simulink library "HeatSourceControl"  (R2025a)
settings: Solver=VariableStepAuto  StartTime=0.0  StopTime=10.0  RelTol=1e-3
libraries: fl_lib x11
settings Model: Creator=vikrants  LastModifiedBy=vikrants

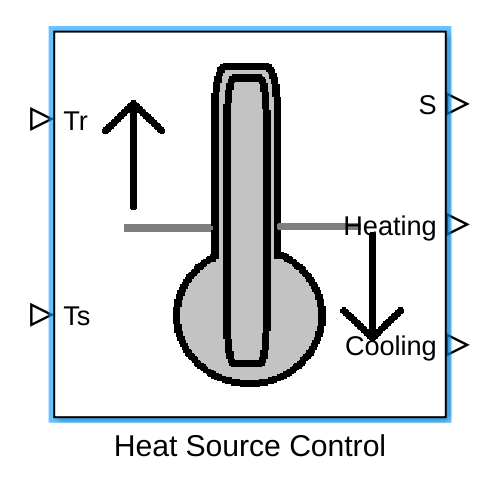
[thumbnail: Simulink's stored preview of the top-level diagram]
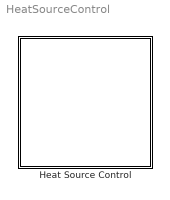
== system HeatSourceControl ==
  Heat Source Control : Subsystem  mask{capacity=12000, num=1, delT=10, tau=1, iniT=280}
      mask prompts: capacity "Heat pump capacity (W)"; num "Number of sources (-)"; delT "Change in water temperature (deg C)"; tau "Measurement time constant (s)"; iniT "Initial water temperature (K)"
      mask Help: web("DocumentationCompositeHeatSourceControl.html")
      mask DialogControl DescGroupVar Prompt: Description
      mask DialogControl DescTextVar Prompt: The block evaluates heating or cooling requirements for a building  based on the measured room temperatures and the specified set point temperature.
      mask DialogControl HeatPump Prompt: Heat Pump
      mask Display: image('HeatSourceControlIcon.png');

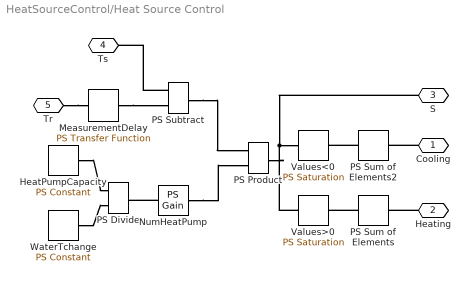
== system HeatSourceControl/Heat Source Control ==
  HeatPumpCapacity : fl_lib/Physical Signals/Sources/PS Constant  constant=capacity J/s
  MeasurementDelay : fl_lib/Physical Signals/Linear Operators/PS Transfer Function  transfer_function_type=foundation.enum.transfer_function_type.lag  T=tau s  T1=2 s  T2=1 s  reset_method=foundation.enum.IntegratorResetSpec.None  initial_condition_spec=foundation.enum.IntegratorICSpec.Internal  y0=iniT K
      settings: InternalSimscapePortConfiguration="{\"Bottom\":[],\"Left\":[{\"id\":\"U\",\"label\":\"\",\"type\":\"input\"}],\"Right\":[{\"id\":\"Y\",\"label\":\"\",\"type\":\"output\"}],\"Top\":[]}"
  NumHeatPump : fl_lib/Physical Signals/Functions/PS Gain  gain=num
  PS Divide : fl_lib/Physical Signals/Functions/PS Divide
  PS Product : fl_lib/Physical Signals/Functions/PS Product
  PS Subtract : fl_lib/Physical Signals/Functions/PS Subtract
  PS Sum of Elements : fl_lib/Physical Signals/Functions/PS Sum of Elements  sumAll=true
      settings: InternalSimscapePortConfiguration="{\"Bottom\":[],\"Left\":[{\"id\":\"I\",\"label\":\"\",\"type\":\"input\"}],\"Right\":[{\"id\":\"O\",\"label\":\"\",\"type\":\"output\"}],\"Top\":[]}"
  PS Sum of Elements2 : fl_lib/Physical Signals/Functions/PS Sum of Elements  sumAll=true
      settings: InternalSimscapePortConfiguration="{\"Bottom\":[],\"Left\":[{\"id\":\"I\",\"label\":\"\",\"type\":\"input\"}],\"Right\":[{\"id\":\"O\",\"label\":\"\",\"type\":\"output\"}],\"Top\":[]}"
  Values<0 : fl_lib/Physical Signals/Nonlinear Operators/PS Saturation  upper_limit=0 J/s  lower_limit=-inf J/s  ZeroCross=true
  Values>0 : fl_lib/Physical Signals/Nonlinear Operators/PS Saturation  upper_limit=inf J/s  lower_limit=0 J/s  ZeroCross=true
  WaterTchange : fl_lib/Physical Signals/Sources/PS Constant  constant=delT K
  Cooling : PMIOPort  Side=Left
  Heating : PMIOPort  Port=2  Side=Left
  S : PMIOPort  Port=3  Side=Left
  Ts : PMIOPort  Port=4  Side=Right
  Tr : PMIOPort  Port=5  Side=Right
  connections:
  PS Subtract/RConn1 -- PS Product/LConn1
  Tr/RConn1 -- MeasurementDelay/LConn1
  PS Subtract/LConn1 -- Ts/RConn1
  Heating/RConn1 -- PS Sum of Elements/RConn1
  Cooling/RConn1 -- PS Sum of Elements2/RConn1
  PS Sum of Elements/LConn1 -- Values>0/RConn1
  PS Sum of Elements2/LConn1 -- Values<0/RConn1
  MeasurementDelay/RConn1 -- PS Subtract/LConn2
  HeatPumpCapacity/RConn1 -- PS Divide/LConn1
  WaterTchange/RConn1 -- PS Divide/LConn2
  NumHeatPump/LConn1 -- PS Divide/RConn1
  NumHeatPump/RConn1 -- PS Product/LConn2
  S/RConn1 -- Values<0/LConn1 -- Values>0/LConn1 -- PS Product/RConn1
